simulink model "slx2_step14_fb-1"  (R2017b)
settings: Solver=ode45  StartTime=0.0  StopTime=10.0  RelTol=1e-3  EnableMultiTasking=on
values from neighbouring files (symbols this model uses):
  A = sys.A    [fn6_state_estimator-1.m]    (also in fn7_feedback-1.m; fn8_obsv_feedback-1.m; main_function-1.m = [a11 a12 a13 a14)
  B = sys.B    [fn6_state_estimator-1.m]    (also in fn7_feedback-1.m; fn8_obsv_feedback-1.m; main_function-1.m = [0)
  C = sys.C    [fn6_state_estimator-1.m]    (also in fn7_feedback-1.m; fn8_obsv_feedback-1.m; main_function-1.m = eye(size(A)))
  D = sys.D    [fn6_state_estimator-1.m]    (also in fn7_feedback-1.m; fn8_obsv_feedback-1.m; main_function-1.m = zeros(size(B)))
  K = place(A, B, P1)    [fn7_feedback-1.m]
  xini = [0;0;0;0]    [main_function-1.m]
settings Model: Creator=mo114c  LastModifiedBy=anusha7
settings DataIOCC: LimitDataPoints=on  SaveFormat=Array
settings OptimizationCC: LifeSpan=inf
settings DebuggingCC: UnderspecifiedInitializationDetection=Classic  MergeDetectMultiDrivingBlocksExec=none  StateNameClashWarn=warning  SFUnexpectedBacktrackingDiag=warning  SFNoUnconditionalDefaultTransitionDiag=warning  SFExecutionAtInitializationDiag=none
settings HardwareCC: ProdBitPerPointer=32  ProdBitPerSizeT=32  ProdBitPerPtrDiffT=32  ProdLargestAtomicFloat=None  ProdIntDivRoundTo=Undefined  ProdEndianess=Unspecified  ProdWordSize=32  ProdHWDeviceType=32-bit Generic
settings ModelReferenceCC: PropagateSignalLabelsOutOfModel=off
settings CodeAppCC: StateflowObjectComments=on
settings GRTTargetCC: TargetLangStandard=C89/C90 (ANSI)  GeneratePreprocessorConditionals=Disable all
settings ConfigComp: CovMetricSettings=dw  CovHtmlReporting=on  CovSaveCumulativeToWorkspaceVar=on  CovSaveSingleToWorkspaceVar=on  CovExternalEMLEnable=off  CovSFcnEnable=off

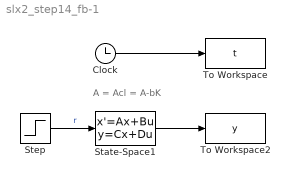
== system slx2_step14_fb-1 ==
  note: A = Acl = A-bK
  Clock : Clock
  State-Space1 : StateSpace  A=A-B*K  B=B  C=C  D=D  InitialCondition=xini
  Step : Step  Time=0  SampleTime=0
  To Workspace : ToWorkspace  VariableName=t  SampleTime=-1
  To Workspace2 : ToWorkspace  VariableName=y  SampleTime=-1
  wires:
  Clock/1 -> To Workspace/1
  State-Space1/1 -> To Workspace2/1
  Step/1 -> State-Space1/1  "r"
